simulink model "DotProduct"  (R2017b)
settings: Solver=FixedStepDiscrete  StartTime=0.0  StopTime=10.0  FixedStep=0.200000  RelTol=1e-3
settings Model: Creator=hbourbou  LastModifiedBy=hbourbou
settings DataIOCC: SaveFormat=StructureWithTime
settings OptimizationCC: LifeSpan=inf
settings DebuggingCC: SFExecutionAtInitializationDiag=none
settings HardwareCC: ProdBitPerSizeT=32  ProdBitPerPtrDiffT=32  ProdWordSize=32  ProdHWDeviceType=Specified
settings CodeAppCC: StateflowObjectComments=on

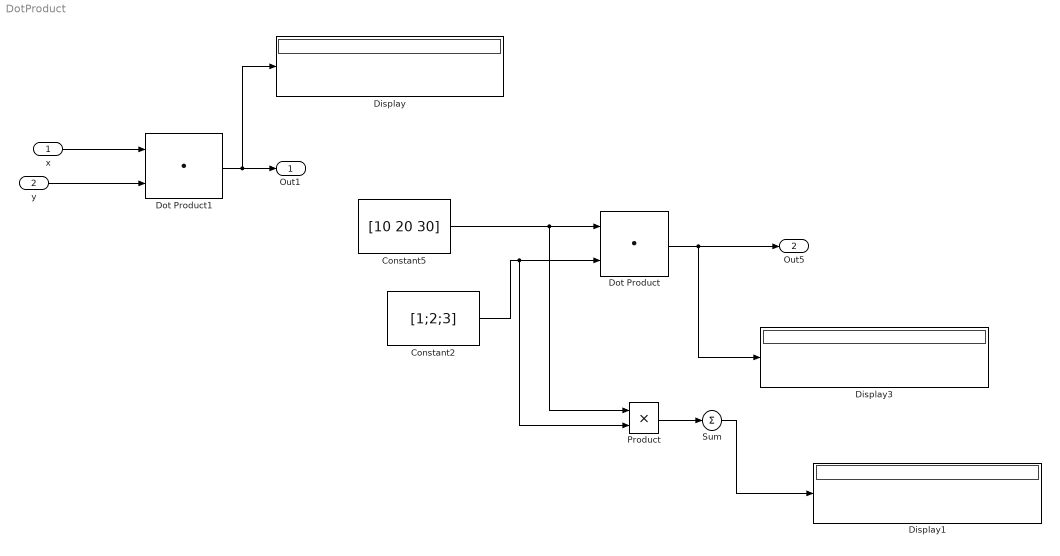
== system DotProduct ==
  x : Inport  OutDataTypeStr=uint8  PortDimensions=3
  y : Inport  Port=2  OutDataTypeStr=uint16
  Constant2 : Constant  Value=[1;2;3]
  Constant5 : Constant  Value=[10 20 30]
  Display : Display
  Display1 : Display
  Display3 : Display
  Dot Product : DotProduct  OutDataTypeStr=int8  InputSameDT=on
  Dot Product1 : DotProduct  OutDataTypeStr=double
  Product : Product
  Sum : Sum  Inputs=1
  Out1 : Outport
  Out5 : Outport  Port=2
  wires:
  Constant2/1 -> Product/2, Dot Product/2
  Dot Product/1 -> Display3/1, Out5/1
  Dot Product1/1 -> Display/1, Out1/1
  x/1 -> Dot Product1/1
  y/1 -> Dot Product1/2
  Constant5/1 -> Product/1, Dot Product/1
  Product/1 -> Sum/1
  Sum/1 -> Display1/1
